simulink model "s_heli_2d_ff_lqr_i"  (Simulink 8.8)
settings: Solver=ode1  StartTime=0.0  StopTime=50  FixedStep=0.001  RelTol=1e-3
values from neighbouring files (symbols this model uses):
  SAT_INT_ERR_PITCH = 5    [setup_lab_heli_2d.m]
  SAT_INT_ERR_YAW = 5    [setup_lab_heli_2d.m]
  Tr_p = 1    [setup_lab_heli_2d.m]
  Tr_y = 1    [setup_lab_heli_2d.m]
undefined symbols (not defined in the file or in its folder): Ki
libraries: simulink x4, simulink_extras x4, heli_2d_lib x3
settings Model: SuppressorTable=22 serialization::archive 11 0 3 0 0 0 0 0  Creator=MLevis  LastModifiedBy=luy0a  ExtModeArmWhenConnect=off
settings OptimizationCC: BooleanDataType=off  OptimizeBlockIOStorage=off  BufferReuse=off  GlobalBufferReuse=off  ExpressionFolding=off  ExpressionDepthLimit=2147483647  LocalBlockOutputs=off  InitFltsAndDblsToZero=on
settings DebuggingCC: SaveWithParameterizedLinksMsg=none  SignalResolutionControl=TryResolveAllWithWarning  SolverPrmCheckMsg=warning  MultiTaskDSMMsg=warning  MultiTaskCondExecSysMsg=none
settings RTWCC: SystemTargetFile=wincon.tlc  MakeCommand=make_wc  TemplateMakefile=wc_default_tmf  Description=WinCon Target
settings STFCustomTargetCC: TargetFcnLib=ansi_tfl_tmw.mat  ModelReferenceCompliant=off  CPPClassGenCompliant=on  SystemTargetFile=wincon.tlc
settings GRTTargetCC: TargetFcnLib=ansi_tfl_tmw.mat  ModelReferenceCompliant=off  ParMdlRefBuildCompliant=off  CompOptLevelCompliant=off  ConcurrentExecutionCompliant=off  GeneratePreprocessorConditionals=Use local settings  MatFileLogging=off  UseToolchainInfoCompliant=off  ExtMode=on  ExtModeTransport=2  ExtModeMexFile=wc_comm
settings CustomProperty: Value=on

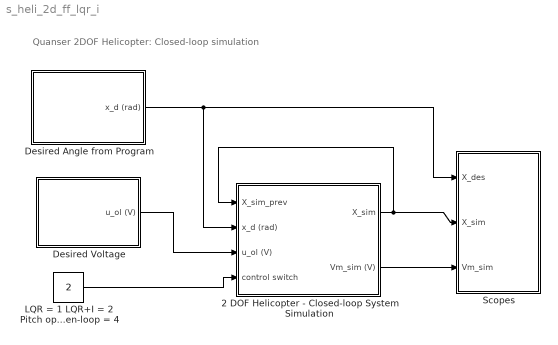
== system s_heli_2d_ff_lqr_i ==
  note: Quanser 2DOF Helicopter: Closed-loop simulation
  2 DOF Helicopter - Closed-loop System Simulation : Subsystem
  Desired Angle from Program : Subsystem
  Desired Voltage : Subsystem
  LQR = 1 LQR+I = 2 Pitch open-loop  = 3 Yaw open-loop = 4 : Constant  Value=2
  Scopes : Subsystem  AncestorBlock=heli_2d_lib/Scopes
  wires:
  2 DOF Helicopter - Closed-loop System Simulation/1(X_sim) -> Scopes/2(X_sim), 2 DOF Helicopter - Closed-loop System Simulation/1(X_sim_prev)
  2 DOF Helicopter - Closed-loop System Simulation/2(Vm_sim (V)) -> Scopes/3(Vm_sim)
  Desired Angle from Program/1(x_d (rad)) -> 2 DOF Helicopter - Closed-loop System Simulation/2(x_d (rad)), Scopes/1(X_des)
  LQR = 1 LQR+I = 2 Pitch open-loop  = 3 Yaw open-loop = 4/1 -> 2 DOF Helicopter - Closed-loop System Simulation/4(control switch)
  Desired Voltage/1(u_ol (V)) -> 2 DOF Helicopter - Closed-loop System Simulation/3(u_ol (V))

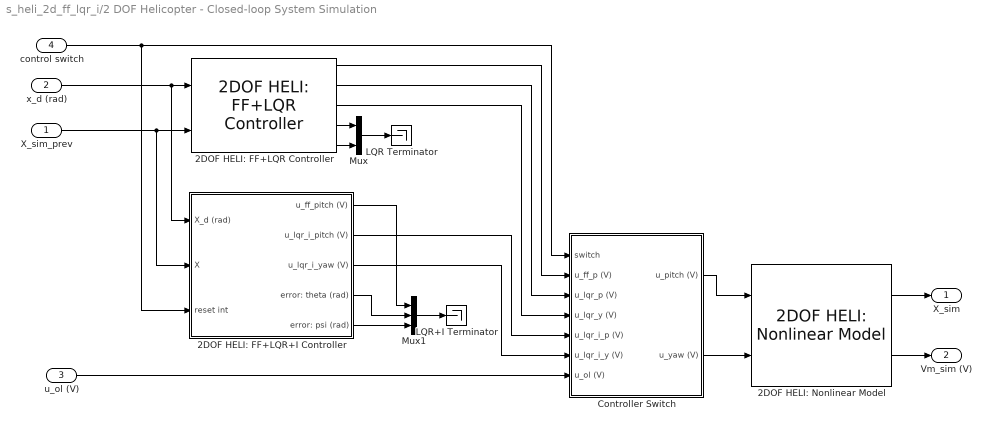
== system s_heli_2d_ff_lqr_i/2 DOF Helicopter - Closed-loop System Simulation ==
  X_sim_prev : Inport
  x_d (rad) : Inport  Port=2
  u_ol (V) : Inport  Port=3
  control switch : Inport  Port=4
  2DOF HELI: FF+LQR Controller : heli_2d_lib/2DOF HELI: FF+LQR Controller
  2DOF HELI: FF+LQR+I Controller : Subsystem  AncestorBlock=heli_2d_lib/2DOF HELI: FF+LQR+I Controller
  2DOF HELI: Nonlinear Model : heli_2d_lib/2DOF HELI: Nonlinear Model
  Controller Switch : Subsystem
  LQR Terminator : Terminator
  LQR+I Terminator : Terminator
  Mux : Mux  Inputs=2
  Mux1 : Mux  Inputs=3
  X_sim : Outport
  Vm_sim (V) : Outport  Port=2
  wires:
  2DOF HELI: Nonlinear Model/1 -> X_sim/1
  2DOF HELI: Nonlinear Model/2 -> Vm_sim (V)/1
  2DOF HELI: FF+LQR Controller/4 -> Mux/1
  2DOF HELI: FF+LQR Controller/5 -> Mux/2
  Mux/1 -> LQR Terminator/1
  Mux1/1 -> LQR+I Terminator/1
  control switch/1 -> 2DOF HELI: FF+LQR+I Controller/3(reset int), Controller Switch/1(switch)
  2DOF HELI: FF+LQR+I Controller/1(u_ff_pitch (V)) -> Mux1/1
  2DOF HELI: FF+LQR+I Controller/2(u_lqr_i_pitch (V)) -> Controller Switch/5(u_lqr_i_p (V))
  2DOF HELI: FF+LQR Controller/3 -> Controller Switch/4(u_lqr_y (V))
  2DOF HELI: FF+LQR Controller/1 -> Controller Switch/2(u_ff_p (V))
  2DOF HELI: FF+LQR Controller/2 -> Controller Switch/3(u_lqr_p (V))
  2DOF HELI: FF+LQR+I Controller/3(u_lqr_i_yaw (V)) -> Controller Switch/6(u_lqr_i_y (V))
  2DOF HELI: FF+LQR+I Controller/4(error: theta (rad)) -> Mux1/2
  2DOF HELI: FF+LQR+I Controller/5(error: psi (rad)) -> Mux1/3
  X_sim_prev/1 -> 2DOF HELI: FF+LQR Controller/2, 2DOF HELI: FF+LQR+I Controller/2(X)
  x_d (rad)/1 -> 2DOF HELI: FF+LQR Controller/1, 2DOF HELI: FF+LQR+I Controller/1(X_d (rad))
  Controller Switch/1(u_pitch (V)) -> 2DOF HELI: Nonlinear Model/1
  Controller Switch/2(u_yaw (V)) -> 2DOF HELI: Nonlinear Model/2
  u_ol (V)/1 -> Controller Switch/7(u_ol (V))

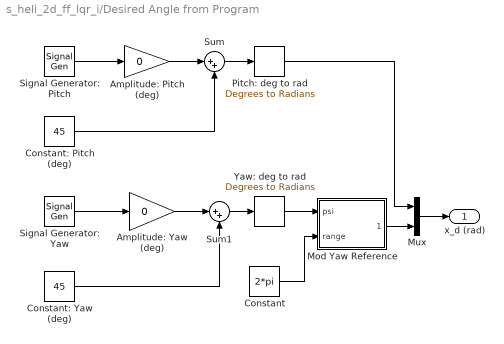
== system s_heli_2d_ff_lqr_i/Desired Angle from Program ==
  Amplitude: Pitch (deg) : Gain  Gain=0
  Amplitude: Yaw (deg) : Gain  Gain=0
  Constant : Constant  Value=2*pi
  Constant: Pitch (deg) : Constant  Value=45
  Constant: Yaw (deg) : Constant  Value=45
  Mod Yaw Reference : Subsystem
  Mux : Mux  Inputs=2
  Pitch: deg to rad : simulink_extras/Transformations/Degrees to Radians
  Signal Generator: Pitch : SignalGenerator  WaveForm=square  Frequency=0.05
  Signal Generator: Yaw : SignalGenerator  WaveForm=square  Frequency=0.05
  Sum : Sum  Inputs=|++
  Sum1 : Sum  Inputs=|++
  Yaw: deg to rad : simulink_extras/Transformations/Degrees to Radians
  x_d (rad) : Outport
  wires:
  Mux/1 -> x_d (rad)/1
  Constant: Yaw (deg)/1 -> Sum1/2
  Amplitude: Yaw (deg)/1 -> Sum1/1
  Signal Generator: Yaw/1 -> Amplitude: Yaw (deg)/1
  Sum1/1 -> Yaw: deg to rad/1
  Constant: Pitch (deg)/1 -> Sum/2
  Amplitude: Pitch (deg)/1 -> Sum/1
  Signal Generator: Pitch/1 -> Amplitude: Pitch (deg)/1
  Sum/1 -> Pitch: deg to rad/1
  Pitch: deg to rad/1 -> Mux/1
  Mod Yaw Reference/1(mod psi) -> Mux/2
  Yaw: deg to rad/1 -> Mod Yaw Reference/1(psi)
  Constant/1 -> Mod Yaw Reference/2(range)

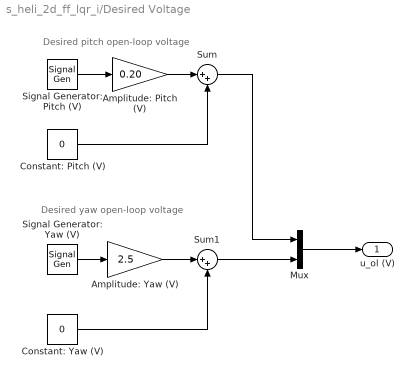
== system s_heli_2d_ff_lqr_i/Desired Voltage ==
  note: Desired yaw open-loop voltage
  note: Desired pitch open-loop voltage
  Amplitude: Pitch (V) : Gain  Gain=0.20
  Amplitude: Yaw (V) : Gain  Gain=2.5
  Constant: Pitch (V) : Constant  Value=0
  Constant: Yaw (V) : Constant  Value=0
  Mux : Mux  Inputs=2
  Signal Generator: Pitch (V) : SignalGenerator  WaveForm=square  Frequency=0.5
  Signal Generator: Yaw (V) : SignalGenerator  WaveForm=square  Frequency=0.01
  Sum : Sum  Inputs=|++
  Sum1 : Sum  Inputs=|++
  u_ol (V) : Outport
  wires:
  Mux/1 -> u_ol (V)/1
  Sum1/1 -> Mux/2
  Sum/1 -> Mux/1
  Signal Generator: Yaw (V)/1 -> Amplitude: Yaw (V)/1
  Amplitude: Yaw (V)/1 -> Sum1/1
  Constant: Yaw (V)/1 -> Sum1/2
  Signal Generator: Pitch (V)/1 -> Amplitude: Pitch (V)/1
  Amplitude: Pitch (V)/1 -> Sum/1
  Constant: Pitch (V)/1 -> Sum/2

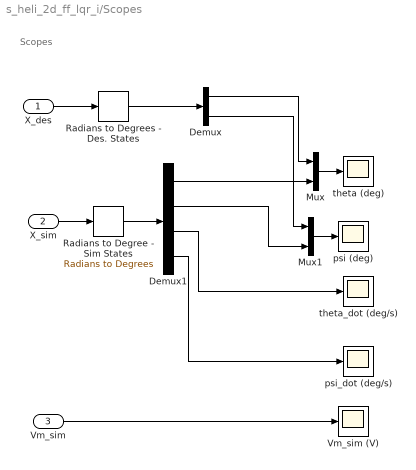
== system s_heli_2d_ff_lqr_i/Scopes ==
  note: Scopes
  X_des : Inport
  X_sim : Inport  Port=2
  Vm_sim : Inport  Port=3
  Demux : Demux  Outputs=2
  Demux1 : Demux
  Mux : Mux  Inputs=2
  Mux1 : Mux  Inputs=2
  Radians to Degree - Sim States : simulink_extras/Transformations/Radians to Degrees
  Radians to Degrees - Des. States : simulink_extras/Transformations/Radians to Degrees
  Vm_sim (V) : Scope
  psi (deg) : Scope
  psi_dot (deg/s) : Scope
  theta (deg) : Scope
  theta_dot (deg/s) : Scope
  wires:
  Demux1/4 -> psi_dot (deg/s)/1
  Demux1/3 -> theta_dot (deg/s)/1
  Mux1/1 -> psi (deg)/1
  Mux/1 -> theta (deg)/1
  Radians to Degree - Sim States/1 -> Demux1/1
  X_sim/1 -> Radians to Degree - Sim States/1
  X_des/1 -> Radians to Degrees - Des. States/1
  Demux/1 -> Mux/1
  Demux1/1 -> Mux/2
  Demux/2 -> Mux1/1
  Demux1/2 -> Mux1/2
  Radians to Degrees - Des. States/1 -> Demux/1
  Vm_sim/1 -> Vm_sim (V)/1

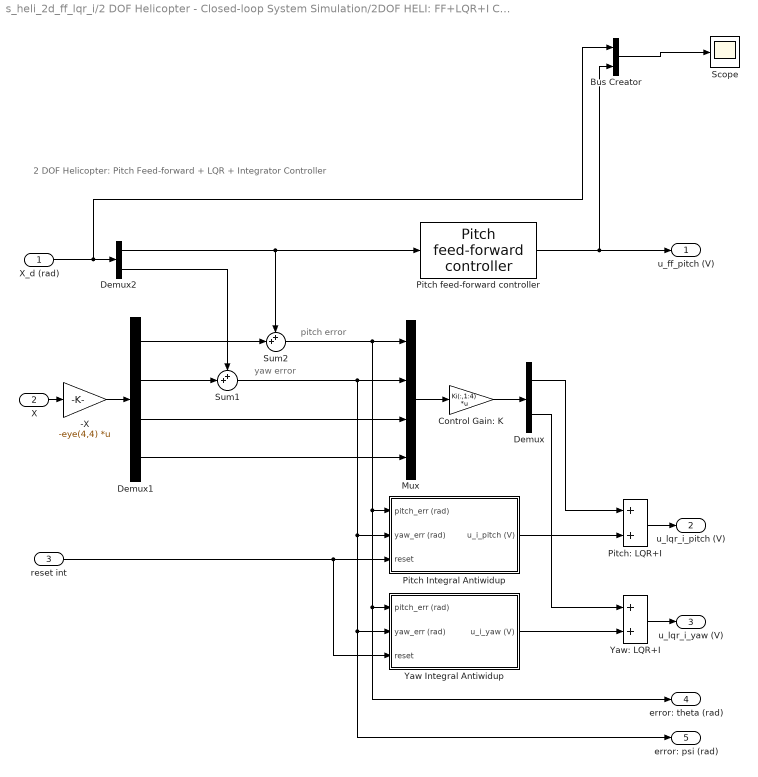
== system s_heli_2d_ff_lqr_i/2 DOF Helicopter - Closed-loop System Simulation/2DOF HELI: FF+LQR+I Controller ==
  note: yaw error
  note: pitch error
  note: 2 DOF Helicopter:
      | Pitch Feed-forward + LQR + Integrator Controller
  X_d (rad) : Inport
  X : Inport  Port=2
  reset int : Inport  Port=3
  -X : Gain  Gain=-eye(4,4)  Multiplication=Matrix(K*u)
  Bus Creator : BusCreator  Inputs=2
  Control Gain: K : Gain  Gain=Ki(:,1:4)  Multiplication=Matrix(K*u)
  Demux : Demux  Outputs=2
  Demux1 : Demux
  Demux2 : Demux  Outputs=2
  Mux : Mux
  Pitch Integral Antiwidup : Subsystem  AncestorBlock=heli_2d_lib/2DOF HELI: FF+LQR+I Controller/Yaw Integral Antiwidup
  Pitch feed-forward controller : heli_2d_lib/Pitch feed-forward controller
  Pitch: LQR+I : Sum
  Scope : Scope
  Sum1 : Sum  Inputs=++|
  Sum2 : Sum  Inputs=++|
  Yaw Integral Antiwidup : Subsystem
  Yaw: LQR+I : Sum
  u_ff_pitch (V) : Outport
  u_lqr_i_pitch (V) : Outport  Port=2
  u_lqr_i_yaw (V) : Outport  Port=3
  error: theta (rad) : Outport  Port=4
  error: psi (rad) : Outport  Port=5
  wires:
  Bus Creator/1 -> Scope/1
  reset int/1 -> Pitch Integral Antiwidup/3(reset), Yaw Integral Antiwidup/3(reset)
  Demux1/2 -> Sum1/2
  Demux2/2 -> Sum1/1
  Demux2/1 -> Sum2/1, Pitch feed-forward controller/1
  X_d (rad)/1 -> Demux2/1, Bus Creator/1
  Yaw Integral Antiwidup/1(u_i_yaw (V)) -> Yaw: LQR+I/2
  Demux/2 -> Yaw: LQR+I/1
  Yaw: LQR+I/1 -> u_lqr_i_yaw (V)/1
  Pitch: LQR+I/1 -> u_lqr_i_pitch (V)/1
  Demux/1 -> Pitch: LQR+I/1
  Pitch Integral Antiwidup/1(u_i_pitch (V)) -> Pitch: LQR+I/2
  Pitch feed-forward controller/1 -> Bus Creator/2, u_ff_pitch (V)/1
  Sum2/1 -> Mux/1, Yaw Integral Antiwidup/1(pitch_err (rad)), error: theta (rad)/1, Pitch Integral Antiwidup/1(pitch_err (rad))
  Demux1/1 -> Sum2/2
  X/1 -> -X/1
  Sum1/1 -> Yaw Integral Antiwidup/2(yaw_err (rad)), error: psi (rad)/1, Pitch Integral Antiwidup/2(yaw_err (rad)), Mux/2
  -X/1 -> Demux1/1
  Control Gain: K/1 -> Demux/1
  Mux/1 -> Control Gain: K/1
  Demux1/3 -> Mux/3
  Demux1/4 -> Mux/4

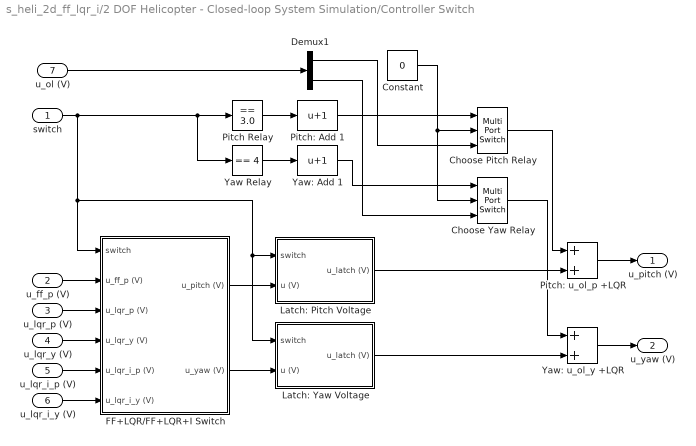
== system s_heli_2d_ff_lqr_i/2 DOF Helicopter - Closed-loop System Simulation/Controller Switch ==
  switch : Inport
  u_ff_p (V) : Inport  Port=2
  u_lqr_p (V) : Inport  Port=3
  u_lqr_y (V) : Inport  Port=4
  u_lqr_i_p (V) : Inport  Port=5
  u_lqr_i_y (V) : Inport  Port=6
  u_ol (V) : Inport  Port=7
  Choose Pitch Relay : MultiPortSwitch  Inputs=2
  Choose Yaw Relay : MultiPortSwitch  Inputs=2
  Constant : Constant  Value=0
  Demux1 : Demux  Outputs=2
  FF+LQR/FF+LQR+I Switch : Subsystem
  Latch: Pitch Voltage : Subsystem
  Latch: Yaw Voltage : Subsystem
  Pitch Relay : simulink/Logic and Bit Operations/Compare To Constant  relop===  const=3.0  OutDataTypeStr=uint8  ZeroCross=off
  Pitch: u_ol_p +LQR : Sum
  Pitch: Add 1 : Bias  Bias=1
  Yaw Relay : simulink/Logic and Bit Operations/Compare To Constant  relop===  const=4  OutDataTypeStr=uint8  ZeroCross=off
  Yaw: u_ol_y +LQR : Sum
  Yaw: Add 1 : Bias  Bias=1
  u_pitch (V) : Outport
  u_yaw (V) : Outport  Port=2
  wires:
  FF+LQR/FF+LQR+I Switch/1(u_pitch (V)) -> Latch: Pitch Voltage/2(u (V))
  FF+LQR/FF+LQR+I Switch/2(u_yaw (V)) -> Latch: Yaw Voltage/2(u (V))
  u_ff_p (V)/1 -> FF+LQR/FF+LQR+I Switch/2(u_ff_p (V))
  u_lqr_p (V)/1 -> FF+LQR/FF+LQR+I Switch/3(u_lqr_p (V))
  u_lqr_y (V)/1 -> FF+LQR/FF+LQR+I Switch/4(u_lqr_y (V))
  u_lqr_i_p (V)/1 -> FF+LQR/FF+LQR+I Switch/5(u_lqr_i_p (V))
  u_lqr_i_y (V)/1 -> FF+LQR/FF+LQR+I Switch/6(u_lqr_i_y (V))
  Latch: Pitch Voltage/1(u_latch (V)) -> Pitch: u_ol_p +LQR/2
  Latch: Yaw Voltage/1(u_latch (V)) -> Yaw: u_ol_y +LQR/2
  switch/1 -> FF+LQR/FF+LQR+I Switch/1(switch), Latch: Pitch Voltage/1(switch), Latch: Yaw Voltage/1(switch), Pitch Relay/1, Yaw Relay/1
  Pitch: u_ol_p +LQR/1 -> u_pitch (V)/1
  Yaw: u_ol_y +LQR/1 -> u_yaw (V)/1
  Pitch Relay/1 -> Pitch: Add 1/1
  Pitch: Add 1/1 -> Choose Pitch Relay/1
  u_ol (V)/1 -> Demux1/1
  Yaw Relay/1 -> Yaw: Add 1/1
  Yaw: Add 1/1 -> Choose Yaw Relay/1
  Constant/1 -> Choose Pitch Relay/2, Choose Yaw Relay/2
  Demux1/1 -> Choose Pitch Relay/3
  Demux1/2 -> Choose Yaw Relay/3
  Choose Yaw Relay/1 -> Yaw: u_ol_y +LQR/1
  Choose Pitch Relay/1 -> Pitch: u_ol_p +LQR/1

== system s_heli_2d_ff_lqr_i/Desired Angle from Program/Mod Yaw Reference ==
  psi : Inport
  range : Inport  Port=2
  Math Function : Math  Operator=mod  SaturateOnIntegerOverflow=on
  Product : Product  RndMeth=Zero
  Sign : Signum
  mod psi : Outport
  wires:
  Product/1 -> Math Function/2
  Sign/1 -> Product/1
  psi/1 -> Math Function/1, Sign/1
  Math Function/1 -> mod psi/1
  range/1 -> Product/2

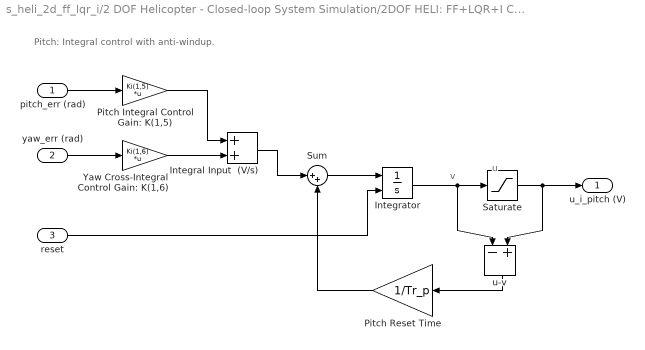
== system s_heli_2d_ff_lqr_i/2 DOF Helicopter - Closed-loop System Simulation/2DOF HELI: FF+LQR+I Controller/Pitch Integral Antiwidup ==
  note: Pitch: Integral control with anti-windup.
  note: v
  note: u
  pitch_err (rad) : Inport
  yaw_err (rad) : Inport  Port=2
  reset : Inport  Port=3
  Integral Input  (V/s) : Sum
  Integrator : Integrator  ExternalReset=rising
  Pitch Integral Control Gain: K(1,5) : Gain  Gain=Ki(1,5)  Multiplication=Matrix(K*u)
  Pitch Reset Time : Gain  Gain=1/Tr_p
  Saturate : Saturate  UpperLimit=SAT_INT_ERR_PITCH  LowerLimit=-SAT_INT_ERR_PITCH
  Sum : Sum  Inputs=|++
  Yaw Cross-Integral Control Gain: K(1,6) : Gain  Gain=Ki(1,6)  Multiplication=Matrix(K*u)
  u-v : Sum  Inputs=-+
  u_i_pitch (V) : Outport
  wires:
  Integral Input  (V/s)/1 -> Sum/1
  Yaw Cross-Integral Control Gain: K(1,6)/1 -> Integral Input  (V/s)/2
  Pitch Integral Control Gain: K(1,5)/1 -> Integral Input  (V/s)/1
  yaw_err (rad)/1 -> Yaw Cross-Integral Control Gain: K(1,6)/1
  reset/1 -> Integrator/2
  Pitch Reset Time/1 -> Sum/2
  Sum/1 -> Integrator/1
  u-v/1 -> Pitch Reset Time/1
  Saturate/1 -> u-v/2, u_i_pitch (V)/1
  Integrator/1 -> Saturate/1, u-v/1
  pitch_err (rad)/1 -> Pitch Integral Control Gain: K(1,5)/1

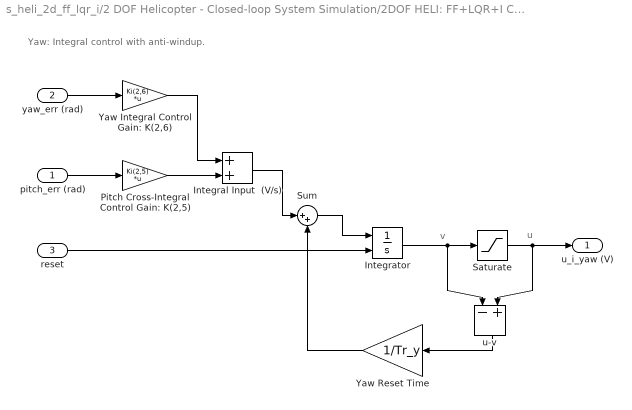
== system s_heli_2d_ff_lqr_i/2 DOF Helicopter - Closed-loop System Simulation/2DOF HELI: FF+LQR+I Controller/Yaw Integral Antiwidup ==
  note: Yaw: Integral control with anti-windup.
  note: u
  note: v
  pitch_err (rad) : Inport
  yaw_err (rad) : Inport  Port=2
  reset : Inport  Port=3
  Integral Input  (V/s) : Sum
  Integrator : Integrator  ExternalReset=rising
  Pitch Cross-Integral Control Gain: K(2,5) : Gain  Gain=Ki(2,5)  Multiplication=Matrix(K*u)
  Saturate : Saturate  UpperLimit=SAT_INT_ERR_YAW  LowerLimit=-SAT_INT_ERR_YAW
  Sum : Sum  Inputs=|++
  Yaw Integral Control Gain: K(2,6) : Gain  Gain=Ki(2,6)  Multiplication=Matrix(K*u)
  Yaw Reset Time : Gain  Gain=1/Tr_y
  u-v : Sum  Inputs=-+
  u_i_yaw (V) : Outport
  wires:
  Integral Input  (V/s)/1 -> Sum/1
  Pitch Cross-Integral Control Gain: K(2,5)/1 -> Integral Input  (V/s)/2
  Yaw Integral Control Gain: K(2,6)/1 -> Integral Input  (V/s)/1
  pitch_err (rad)/1 -> Pitch Cross-Integral Control Gain: K(2,5)/1
  reset/1 -> Integrator/2
  yaw_err (rad)/1 -> Yaw Integral Control Gain: K(2,6)/1
  Integrator/1 -> u-v/1, Saturate/1
  Saturate/1 -> u_i_yaw (V)/1, u-v/2
  u-v/1 -> Yaw Reset Time/1
  Sum/1 -> Integrator/1
  Yaw Reset Time/1 -> Sum/2

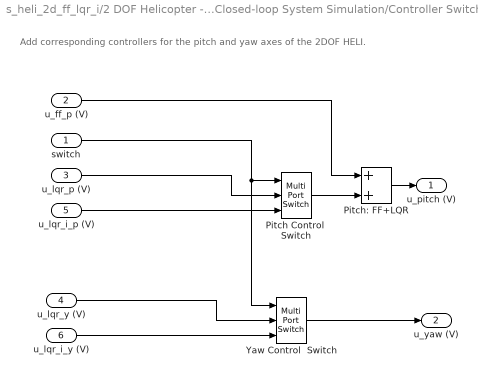
== system s_heli_2d_ff_lqr_i/2 DOF Helicopter - Closed-loop System Simulation/Controller Switch/FF+LQR/FF+LQR+I Switch ==
  note: Add corresponding controllers for the pitch and yaw axes of the 2DOF HELI.
  switch : Inport
  u_ff_p (V) : Inport  Port=2
  u_lqr_p (V) : Inport  Port=3
  u_lqr_y (V) : Inport  Port=4
  u_lqr_i_p (V) : Inport  Port=5
  u_lqr_i_y (V) : Inport  Port=6
  Pitch Control  Switch : MultiPortSwitch  Inputs=2
  Pitch: FF+LQR : Sum
  Yaw Control  Switch : MultiPortSwitch  Inputs=2
  u_pitch (V) : Outport
  u_yaw (V) : Outport  Port=2
  wires:
  Pitch Control  Switch/1 -> Pitch: FF+LQR/2
  u_ff_p (V)/1 -> Pitch: FF+LQR/1
  Pitch: FF+LQR/1 -> u_pitch (V)/1
  u_lqr_p (V)/1 -> Pitch Control  Switch/2
  u_lqr_y (V)/1 -> Yaw Control  Switch/2
  Yaw Control  Switch/1 -> u_yaw (V)/1
  u_lqr_i_p (V)/1 -> Pitch Control  Switch/3
  u_lqr_i_y (V)/1 -> Yaw Control  Switch/3
  switch/1 -> Pitch Control  Switch/1, Yaw Control  Switch/1

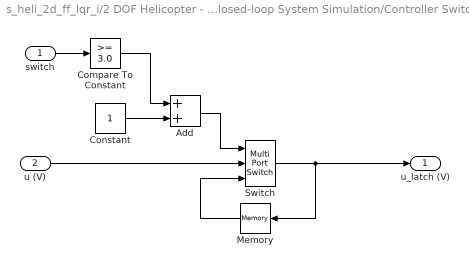
== system s_heli_2d_ff_lqr_i/2 DOF Helicopter - Closed-loop System Simulation/Controller Switch/Latch: Pitch Voltage ==
  switch : Inport
  u (V) : Inport  Port=2
  Add : Sum
  Compare To Constant : simulink/Logic and Bit Operations/Compare To Constant  relop=>=  const=3.0  OutDataTypeStr=uint8  ZeroCross=off
  Constant : Constant
  Memory : Memory
  Switch : MultiPortSwitch  Inputs=2
  u_latch (V) : Outport
  wires:
  Switch/1 -> Memory/1, u_latch (V)/1
  Memory/1 -> Switch/3
  Add/1 -> Switch/1
  u (V)/1 -> Switch/2
  switch/1 -> Compare To Constant/1
  Compare To Constant/1 -> Add/1
  Constant/1 -> Add/2

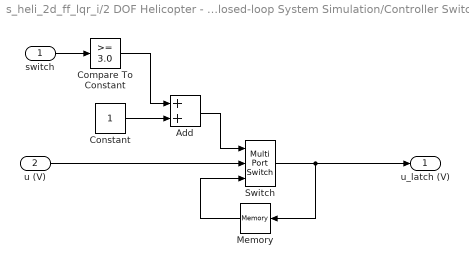
== system s_heli_2d_ff_lqr_i/2 DOF Helicopter - Closed-loop System Simulation/Controller Switch/Latch: Yaw Voltage ==
  switch : Inport
  u (V) : Inport  Port=2
  Add : Sum
  Compare To Constant : simulink/Logic and Bit Operations/Compare To Constant  relop=>=  const=3.0  OutDataTypeStr=uint8  ZeroCross=off
  Constant : Constant
  Memory : Memory
  Switch : MultiPortSwitch  Inputs=2
  u_latch (V) : Outport
  wires:
  Constant/1 -> Add/2
  Compare To Constant/1 -> Add/1
  switch/1 -> Compare To Constant/1
  u (V)/1 -> Switch/2
  Add/1 -> Switch/1
  Memory/1 -> Switch/3
  Switch/1 -> u_latch (V)/1, Memory/1
